simulink model "stateflow_History_Junction"  (R2025b)
settings: Solver=FixedStepDiscrete  StartTime=0.0  StopTime=10.0  FixedStep=0.01  RelTol=1e-3
libraries: simulink x1
settings Model: Creator=soura  LastModifiedBy=soura

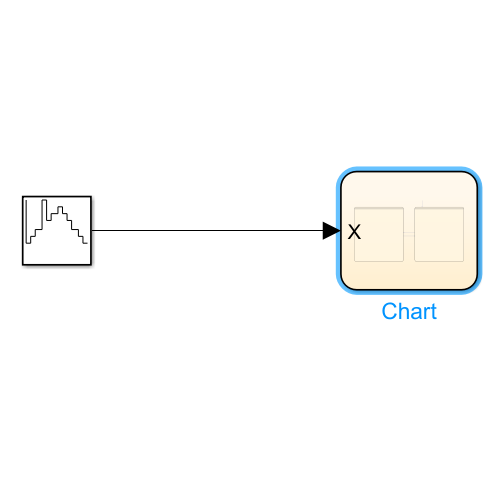
[thumbnail: Simulink's stored preview of the top-level diagram]
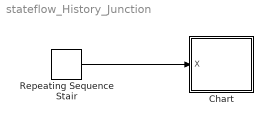
== system stateflow_History_Junction ==
  Chart : Stateflow chart  TreatAsAtomicUnit=on
  Repeating Sequence Stair : simulink/Sources/Repeating Sequence Stair  OutValues=[1 2 3 7 4 5 6 5 4 3 2 1].'  tsamp=-1  OutMin=[]  OutMax=[]  OutDataTypeStr=double  OutputDataTypeScalingMode=double  OutDataType=fixdt(0,8)  ConRadixGroup=Best Precision: Vector-wise  OutScaling=2^-12
  wires:
  Repeating Sequence Stair/1 -> Chart/1(X)

== stateflow chart stateflow_History_Junction/Chart ==
  settings: executeAtInitialization=1
  state Child1
    state On
    state Off
    state low
    (default) -> Child1.On
    Child1.On -> Child1.Off
    Child1.Off -> Child1.On [order 2]
    Child1.Off -> Child1.low [order 1]
    Child1.low -> Child1.Off
  state Child
    (history)
    state On
    state Off
    state low
    (default) -> Child.On
    Child.On -> Child.Off : [X==1]
    Child.Off -> Child.On [order 2] : [X==4]
    Child.Off -> Child.low [order 1] : [X==2]
    Child.low -> Child.Off : [X==3]
  (default) -> Child
  Child -> Child1 : [X>5]
  Child1 -> Child : [X<5]
  data: X input
